simulink model "BRGH_MRAC_simulink"  (R2023b)
settings: Solver=VariableStepAuto  StartTime=0.0  StopTime=simTime  RelTol=1e-3
values from neighbouring files (symbols this model uses):
  alpha = 1    [MRAC_script.m]
  freq1 = .2    (= 0.2)    [MRAC_script.m]
  freq2 = .23    (= 0.23)    [MRAC_script.m]
  freq3 = .5    (= 0.5)    [MRAC_script.m]
  gamma = 1    [MRAC_script.m]
  km = 1    [MRAC_script.m]
  kp = b1    (= 0.3)    [MRAC_script.m]
  Lambda0 = [1 lambda0]    [MRAC_script.m]
  r1 = 1.2    [MRAC_script.m]
  r2 = 1    [MRAC_script.m]
  r3 = .5    (= 0.5)    [MRAC_script.m]
  Rm = [1 0.1]    [MRAC_script.m]
  Rp = [1 a1 a0]    [MRAC_script.m]
  theta_bar = S\p    [MRAC_script.m]
  Zm = 1    [MRAC_script.m]
  Zp = [0 1 b0/b1]    [MRAC_script.m]
settings Model: Creator=eliasoa  LastModifiedBy=eliasoa

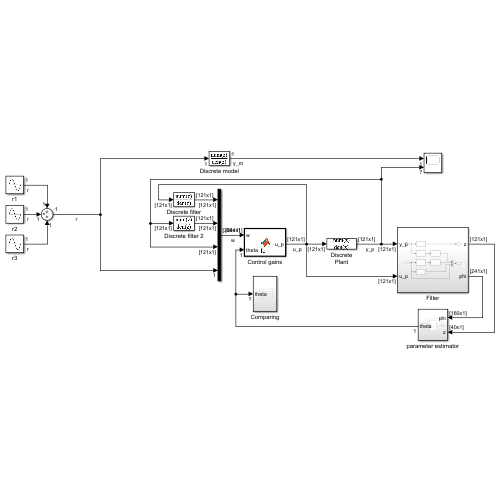
[thumbnail: Simulink's stored preview of the top-level diagram]
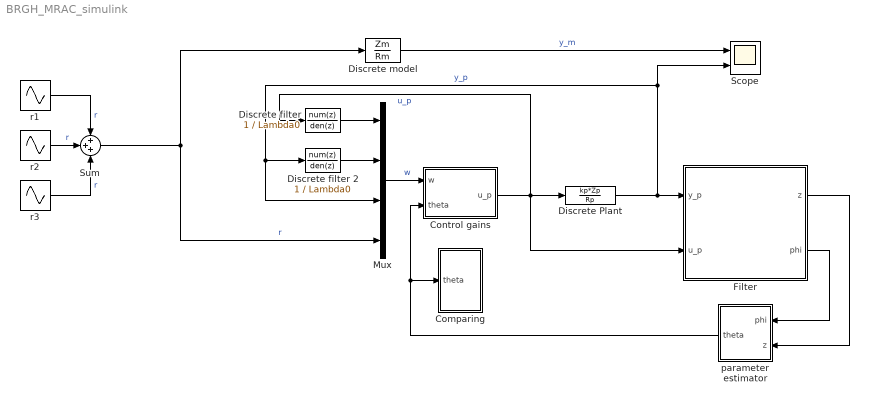
== system BRGH_MRAC_simulink ==
  Comparing : Subsystem
  Control gains : MATLAB Function  TreatAsAtomicUnit=on
  Discrete Plant : DiscreteTransferFcn  Numerator=kp*Zp  Denominator=Rp
  Discrete filter : DiscreteTransferFcn  Numerator=1  Denominator=Lambda0
  Discrete filter 2 : DiscreteTransferFcn  Numerator=1  Denominator=Lambda0
  Discrete model : DiscreteTransferFcn  Numerator=Zm  Denominator=Rm
  Filter : Subsystem
  Mux : Mux
  Scope : Scope  NumInputPorts=2
  Sum : Sum  Inputs=+++
  parameter estimator : Subsystem
  r1 : Sin  Amplitude=r1  Frequency=freq1  SampleTime=0
  r2 : Sin  Amplitude=r2  Frequency=freq2  SampleTime=0
  r3 : Sin  Amplitude=r3  Frequency=freq3  SampleTime=0
  wires:
  Discrete model/1 -> Scope/1  "y_m"
  Mux/1 -> Control gains/1(w)  "w"
  Discrete Plant/1 -> Scope/2, Mux/3, Discrete filter 2/1, Filter/1(y_p)  "y_p"
  Control gains/1(u_p) -> Discrete filter/1, Discrete Plant/1, Filter/2(u_p)  "u_p"
  Discrete filter 2/1 -> Mux/2
  Discrete filter/1 -> Mux/1
  Filter/1(z) -> parameter estimator/2(z)
  Filter/2(phi) -> parameter estimator/1(phi)
  parameter estimator/1(theta) -> Control gains/2(theta), Comparing/1(theta)
  r1/1 -> Sum/1  "r"
  Sum/1 -> Discrete model/1, Mux/4  "r"
  r2/1 -> Sum/2  "r"
  r3/1 -> Sum/3  "r"

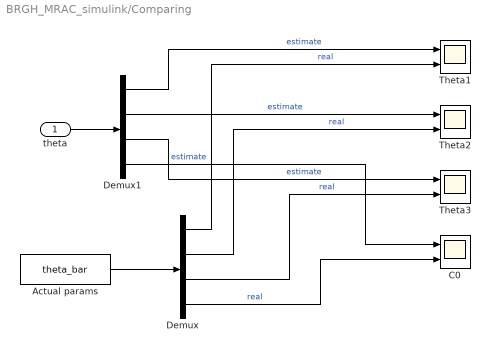
== system BRGH_MRAC_simulink/Comparing ==
  theta : Inport
  Actual params : Constant  Value=theta_bar
  C0 : Scope  NumInputPorts=2
  Demux : Demux
  Demux1 : Demux
  Theta1 : Scope  NumInputPorts=2
  Theta2 : Scope  NumInputPorts=2
  Theta3 : Scope  NumInputPorts=2
  wires:
  Actual params/1 -> Demux/1
  theta/1 -> Demux1/1
  Demux1/1 -> Theta1/1  "estimate"
  Demux/1 -> Theta1/2  "real"
  Demux1/2 -> Theta2/1  "estimate"
  Demux/2 -> Theta2/2  "real"
  Demux1/3 -> Theta3/1  "estimate"
  Demux/3 -> Theta3/2  "real"
  Demux1/4 -> C0/1  "estimate"
  Demux/4 -> C0/2  "real"

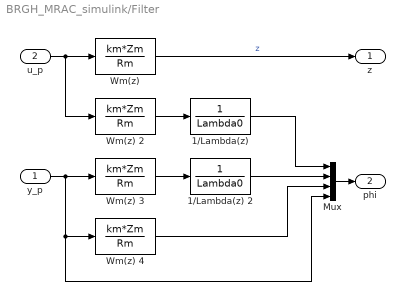
== system BRGH_MRAC_simulink/Filter ==
  y_p : Inport
  u_p : Inport  Port=2
  1/Lambda(z) : DiscreteTransferFcn  Numerator=1  Denominator=Lambda0
  1/Lambda(z) 2 : DiscreteTransferFcn  Numerator=1  Denominator=Lambda0
  Mux : Mux
  Wm(z) : DiscreteTransferFcn  Numerator=km*Zm  Denominator=Rm
  Wm(z) 2 : DiscreteTransferFcn  Numerator=km*Zm  Denominator=Rm
  Wm(z) 3 : DiscreteTransferFcn  Numerator=km*Zm  Denominator=Rm
  Wm(z) 4 : DiscreteTransferFcn  Numerator=km*Zm  Denominator=Rm
  z : Outport
  phi : Outport  Port=2
  wires:
  Wm(z)/1 -> z/1  "z"
  u_p/1 -> Wm(z) 2/1, Wm(z)/1
  Wm(z) 2/1 -> 1/Lambda(z)/1
  y_p/1 -> Wm(z) 3/1, Wm(z) 4/1, Mux/4
  Wm(z) 3/1 -> 1/Lambda(z) 2/1
  1/Lambda(z)/1 -> Mux/1
  Wm(z) 4/1 -> Mux/3
  Mux/1 -> phi/1
  1/Lambda(z) 2/1 -> Mux/2

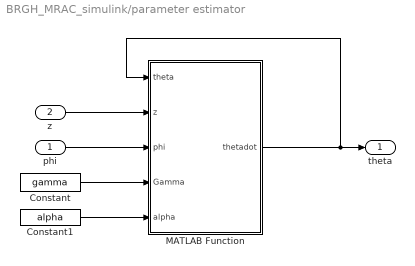
== system BRGH_MRAC_simulink/parameter estimator ==
  phi : Inport
  z : Inport  Port=2
  Constant : Constant  Value=gamma
  Constant1 : Constant  Value=alpha
  MATLAB Function : MATLAB Function  TreatAsAtomicUnit=on
  theta : Outport
  wires:
  Constant1/1 -> MATLAB Function/5(alpha)
  MATLAB Function/1(thetadot) -> theta/1, MATLAB Function/1(theta)
  phi/1 -> MATLAB Function/3(phi)
  z/1 -> MATLAB Function/2(z)
  Constant/1 -> MATLAB Function/4(Gamma)

== matlab function BRGH_MRAC_simulink/Control gains ==
  data: w input; theta input; u_p output
function u_p = fcn(w,theta)

u_p = theta'*w;

== matlab function BRGH_MRAC_simulink/parameter estimator/MATLAB Function ==
  data: theta input; thetadot output; z input; phi input; Gamma input; alpha input
function thetadot = fcn(theta,z,phi,Gamma,alpha)
m2 = 1 + alpha*(phi'*phi);
epsilon = (z-theta'*phi)/m2;
thetadot = Gamma * epsilon * phi;
